simulink library "CryoDetLibCMB"  (R2016b)
settings: Solver=VariableStepAuto  StartTime=0.0  StopTime=10.0  RelTol=1e-3
undefined symbols (not defined in the file): Fclk, xlipgetpartsetting
libraries: xbsIndex_r4 x329, CryoDetLibCMB x20, CryoDetLib x2, simulink x1
(part 1 of 3)
settings Model: Creator=ssmith  LastModifiedBy=ssmith

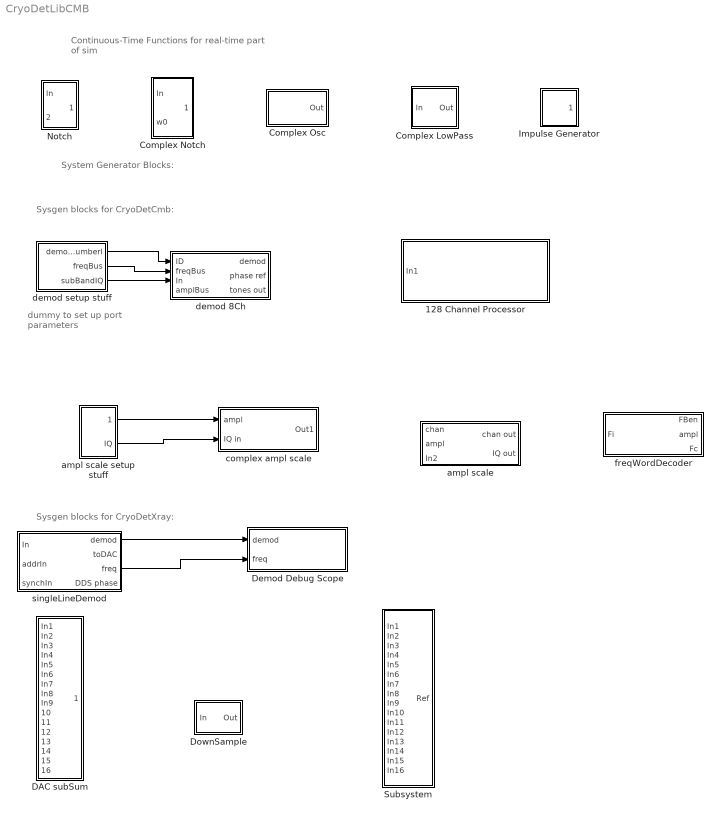
== system CryoDetLibCMB ==
  note: dummy to set up port parameters
  note: Sysgen blocks for CryoDetXray:
  note: Continuous-Time Functions
      | for real-time part of sim
  note: System Generator Blocks:
  note: Sysgen blocks for CryoDetCmb:
  128 Channel Processor : Subsystem
  Complex LowPass : Subsystem  mask{num=0, den=0}
  Complex Notch : Subsystem  mask(Complex Notch Filter){Q=10, depth=1, Q1=10, depth1=1, Q2=10, depth2=1}
      mask help: Specify w0, Q, and notch depth (1 is max depth, 0 is no notch)
      mask init:
      | Q1 = Q
      | depth1 = depth
      | Q2 = Q
      | depth2 = depth
      mask TypeOptions Q1: Notch1/Q
      mask TypeOptions depth1: Notch1/depth
      mask TypeOptions Q2: Notch2/Q
      mask TypeOptions depth2: Notch2/depth
  Complex Osc : Subsystem  mask{Freq=40e6, Ampl=0.2}
  DAC subSum : Subsystem
  Demod Debug Scope : Subsystem
  DownSample : Subsystem
  Impulse Generator : Subsystem  mask(Impulse Generator){Impulse=0, width=0, Period=0, delay=0}
      mask help:
      | Generate an psuedo-impulse via a rectangular pulse of amplitude given impulse/width so time intagral is impulse
      | repeating at period given by parameter Period starting at time "delay"
  Notch : Subsystem  mask(Notch filter){Q=10, depth=1}
      mask help:
      | Continuous-time notch filter acting in input with input parameters:
      | w0	center frequency
      | Q	center frequency/bandwidth
      | depth	depth of notch: 0==> no notch, 1 ==> deep notch
  Subsystem : Subsystem
  ampl scale : Subsystem
  ampl scale setup stuff : Subsystem
  complex ampl scale : Subsystem
  demod 8Ch : Subsystem
  demod setup stuff : Subsystem
  freqWordDecoder : Subsystem
  singleLineDemod : Subsystem
  wires:
  singleLineDemod/3(freq) -> Demod Debug Scope/2(freq)
  singleLineDemod/1(demod) -> Demod Debug Scope/1(demod)
  demod setup stuff/3(subBandIQ) -> demod 8Ch/3(In)
  demod setup stuff/1(demod numberl) -> demod 8Ch/1(ID)
  demod setup stuff/2(freqBus) -> demod 8Ch/2(freqBus)
  ampl scale setup stuff/1(ampl) -> complex ampl scale/1(ampl)
  ampl scale setup stuff/2(IQ) -> complex ampl scale/2(IQ in)

== system CryoDetLibCMB/128 Channel Processor ==
  note: dF using CORIDC rotation
      | added 11/14/17
  note: 128 Channel Processor
      | Contains baeband tone generator
      | demodulator
      | resonator frequency error estimator
      | loop filter
  In1 : Inport
  128 Channel Demodulator : Subsystem
  Loop Filter : Subsystem
  dF1 : Subsystem
  wires:
  In1/1 -> 128 Channel Demodulator/1(in)
  dF1/1(dF) -> Loop Filter/1(In2)
  128 Channel Demodulator/1(demod) -> dF1/1(demod)
  Loop Filter/1(Out2) -> 128 Channel Demodulator/2(freqBus)
  128 Channel Demodulator/2(phase ref out) -> dF1/2(ref phase)

== system CryoDetLibCMB/Complex LowPass ==
  note: Apply continuous-time transfer function given by num/den to complex continuous-time signal
  In : Inport
  Complex to Real-Imag : ComplexToRealImag
  Real-Imag to Complex : RealImagToComplex
  Transfer Fcn : TransferFcn  Numerator=num  Denominator=den
  Transfer Fcn1 : TransferFcn  Numerator=num  Denominator=den
  Out : Outport
  wires:
  Complex to Real-Imag/2 -> Transfer Fcn1/1
  Transfer Fcn1/1 -> Real-Imag to Complex/2
  In/1 -> Complex to Real-Imag/1
  Real-Imag to Complex/1 -> Out/1
  Transfer Fcn/1 -> Real-Imag to Complex/1
  Complex to Real-Imag/1 -> Transfer Fcn/1

== system CryoDetLibCMB/Complex Notch ==
  In : Inport
  w0 : Inport  Port=2
  Complex to Real-Imag : ComplexToRealImag
  Notch1 : CryoDetLib/Notch  Q=Q1  depth=depth1
  Notch2 : CryoDetLib/Notch  Q=Q2  depth=depth2
  Real-Imag to Complex : RealImagToComplex
  Out : Outport
  wires:
  Complex to Real-Imag/2 -> Notch2/1
  Notch2/1 -> Real-Imag to Complex/2
  In/1 -> Complex to Real-Imag/1
  Real-Imag to Complex/1 -> Out/1
  Notch1/1 -> Real-Imag to Complex/1
  w0/1 -> Notch2/2, Notch1/2
  Complex to Real-Imag/1 -> Notch1/1

== system CryoDetLibCMB/Complex Osc ==
  Cosine : Sin  Amplitude=Ampl  Frequency=2*pi*Freq  Phase=pi/2  SampleTime=0
  Real-Imag to Complex : RealImagToComplex
  Sine : Sin  Amplitude=Ampl  Frequency=2*pi*Freq  SampleTime=0
  Out : Outport
  wires:
  Real-Imag to Complex/1 -> Out/1
  Cosine/1 -> Real-Imag to Complex/1
  Sine/1 -> Real-Imag to Complex/2

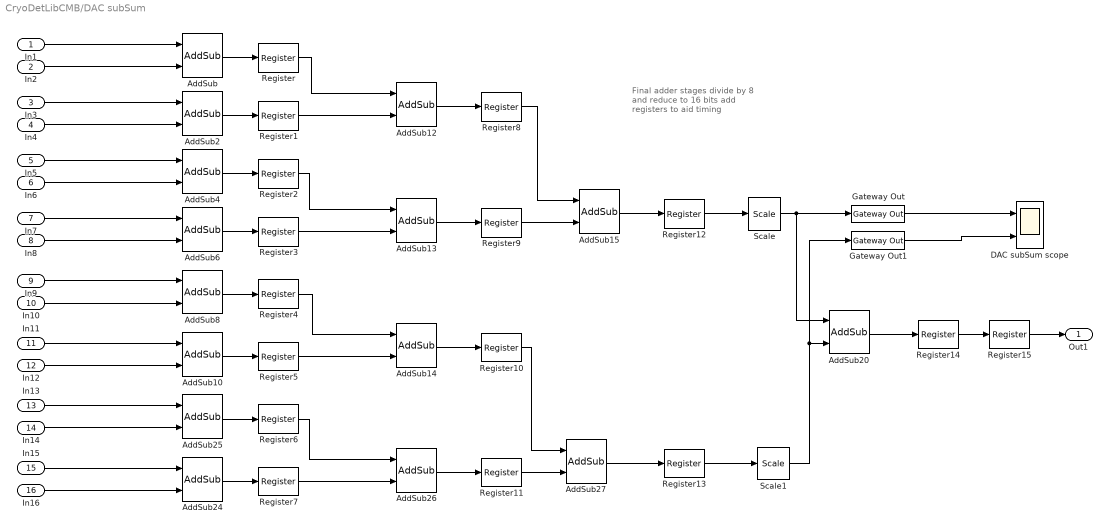
== system CryoDetLibCMB/DAC subSum ==
  note: Final adder stages
      | divide by 8
      | and reduce to 16 bits
      | add registers to aid timing
  In1 : Inport
  In2 : Inport  Port=2
  In3 : Inport  Port=3
  In4 : Inport  Port=4
  In5 : Inport  Port=5
  In6 : Inport  Port=6
  In7 : Inport  Port=7
  In8 : Inport  Port=8
  In9 : Inport  Port=9
  In10 : Inport  Port=10
  In11 : Inport  Port=11
  In12 : Inport  Port=12
  In13 : Inport  Port=13
  In14 : Inport  Port=14
  In15 : Inport  Port=15
  In16 : Inport  Port=16
  AddSub{,2,4,6,8,10,12..15,24..27} (14 alike) : xbsIndex_r4/AddSub  mode=Addition  use_carryin=off  use_carryout=off  en=off  latency=3  precision=User Defined  arith_type="Signed  (2's comp)"  n_bits=20  bin_pt=15  quantization=Truncate  overflow=Wrap  use_behavioral_HDL=off  hw_selection=Fabric  pipelined=off  dbl_ovrd=off  block_type=addsub
  AddSub20 : xbsIndex_r4/AddSub  mode=Addition  use_carryin=off  use_carryout=off  en=off  latency=3  precision=User Defined  arith_type="Signed  (2's comp)"  n_bits=16  bin_pt=15  quantization="Round  (unbiased: +/- Inf)"  overflow=Saturate  use_behavioral_HDL=off  hw_selection=Fabric  pipelined=off  dbl_ovrd=off  block_type=addsub
  DAC subSum scope : Scope  NumInputPorts=2
  Gateway Out : xbsIndex_r4/Gateway Out  inherit_from_input=off  hdl_port=off  rows=1  columns=1  UseAsDAC=off  DACChannel='1'  interface=None  automatic_assignment=on  address_offset=hex2dec('00')  intf_name=''  intf_description=''  timing_constraint=None  locs_specified=off  LOCs={}  io_standard={}  block_type=gatewayout
  Gateway Out1 : xbsIndex_r4/Gateway Out  inherit_from_input=off  hdl_port=off  rows=1  columns=1  UseAsDAC=off  DACChannel='1'  interface=None  automatic_assignment=on  address_offset=hex2dec('00')  intf_name=''  intf_description=''  timing_constraint=None  locs_specified=off  LOCs={}  io_standard={}  block_type=gatewayout
  Register{,1..15} (16 alike) : xbsIndex_r4/Register  init=0  rst=off  en=off  dbl_ovrd=off  block_type=register
  Scale : xbsIndex_r4/Scale  scale_factor=-3  dbl_ovrd=off  block_type=scale
  Scale1 : xbsIndex_r4/Scale  scale_factor=-3  dbl_ovrd=off  block_type=scale
  Out1 : Outport
  wires:
  AddSub20/1 -> Register14/1
  AddSub/1 -> Register/1
  AddSub2/1 -> Register1/1
  AddSub4/1 -> Register2/1
  AddSub6/1 -> Register3/1
  AddSub8/1 -> Register4/1
  AddSub10/1 -> Register5/1
  AddSub12/1 -> Register8/1
  AddSub13/1 -> Register9/1
  AddSub15/1 -> Register12/1
  In1/1 -> AddSub/1
  Scale/1 -> Gateway Out/1, AddSub20/1
  Scale1/1 -> Gateway Out1/1, AddSub20/2
  AddSub25/1 -> Register6/1
  AddSub24/1 -> Register7/1
  AddSub14/1 -> Register10/1
  AddSub27/1 -> Register13/1
  AddSub26/1 -> Register11/1
  In16/1 -> AddSub24/2
  In15/1 -> AddSub24/1
  In14/1 -> AddSub25/2
  In13/1 -> AddSub25/1
  In12/1 -> AddSub10/2
  In11/1 -> AddSub10/1
  In10/1 -> AddSub8/2
  In9/1 -> AddSub8/1
  In7/1 -> AddSub6/1
  In6/1 -> AddSub4/2
  In5/1 -> AddSub4/1
  In4/1 -> AddSub2/2
  In3/1 -> AddSub2/1
  In2/1 -> AddSub/2
  In8/1 -> AddSub6/2
  Gateway Out1/1 -> DAC subSum scope/2
  Gateway Out/1 -> DAC subSum scope/1
  Register/1 -> AddSub12/1
  Register1/1 -> AddSub12/2
  Register2/1 -> AddSub13/1
  Register3/1 -> AddSub13/2
  Register4/1 -> AddSub14/1
  Register5/1 -> AddSub14/2
  Register6/1 -> AddSub26/1
  Register7/1 -> AddSub26/2
  Register8/1 -> AddSub15/1
  Register9/1 -> AddSub15/2
  Register10/1 -> AddSub27/1
  Register11/1 -> AddSub27/2
  Register12/1 -> Scale/1
  Register13/1 -> Scale1/1
  Register14/1 -> Register15/1
  Register15/1 -> Out1/1

== system CryoDetLibCMB/Demod Debug Scope ==
  note: Debug Demodulation
  demod : Inport
  freq : Inport  Port=2
  Complex to Magnitude-Angle : ComplexToMagnitudeAngle  Output=Magnitude
  Demux1 : Demux
  Gain : Gain  Gain=Fclk
  Gateway Out{1,3..6} (5 alike) : xbsIndex_r4/Gateway Out  inherit_from_input=off  hdl_port=off  rows=1  columns=1  UseAsDAC=off  DACChannel='1'  interface=None  automatic_assignment=on  address_offset=hex2dec('00')  intf_name=''  intf_description=''  timing_constraint=None  locs_specified=off  LOCs={}  io_standard={}  block_type=gatewayout
  Mux4 : Mux  Inputs=3
  Mux5 : Mux  Inputs=2
  Real-Imag to Complex : RealImagToComplex
  block downconverter Scope : Scope  NumInputPorts=3
  wires:
  demod/1 -> Demux1/1
  Demux1/1 -> Gateway Out3/1
  Demux1/2 -> Gateway Out4/1
  Demux1/3 -> Gateway Out5/1
  Demux1/4 -> Gateway Out6/1
  Gateway Out6/1 -> Mux5/2
  Gateway Out5/1 -> Mux5/1
  Gateway Out4/1 -> Mux4/2, Real-Imag to Complex/1
  Gateway Out3/1 -> Mux4/1, Real-Imag to Complex/2
  Mux4/1 -> block downconverter Scope/1
  Mux5/1 -> block downconverter Scope/2
  Complex to Magnitude-Angle/1 -> Mux4/3
  Real-Imag to Complex/1 -> Complex to Magnitude-Angle/1
  freq/1 -> Gateway Out1/1
  Gateway Out1/1 -> Gain/1
  Gain/1 -> block downconverter Scope/3

== system CryoDetLibCMB/DownSample ==
  note: DownSample with rate change given by Naxi
  In : Inport
  Down Sample : xbsIndex_r4/Down Sample  sample_ratio=Naxi  sample_phase="Last Value of Frame  (most efficient)"  en=off  rst=off  latency=1  dbl_ovrd=off  block_type=dsamp
  Register : xbsIndex_r4/Register  init=0  rst=off  en=off  dbl_ovrd=off  block_type=register
  Register1 : xbsIndex_r4/Register  init=0  rst=off  en=off  dbl_ovrd=off  block_type=register
  Out : Outport
  wires:
  Register/1 -> Register1/1
  In/1 -> Down Sample/1
  Down Sample/1 -> Register/1
  Register1/1 -> Out/1

== system CryoDetLibCMB/Impulse Generator ==
  note: Parameters are:
      | width:	 pulse width (seconds)
      | Impulse:	Area of pulse = Amplitude*width
      | Period:	Pulse repetition time (seconds)
      | delay:	start time of pulse (seconds)
  Pulse Generator1 : DiscretePulseGenerator  PulseType=Time based  Amplitude=Impulse/width  Period=Period  PulseWidth=100 * width/Period  PhaseDelay=delay
  Out1 : Outport
  wires:
  Pulse Generator1/1 -> Out1/1

== system CryoDetLibCMB/Notch ==
  note: Notch Filter with center angular frequency w0, finite Q, and notch depth
  In : Inport
  w0 : Inport  Port=2
  Gain : Gain  Gain=depth
  Gain1 : Gain  Gain=1/Q
  Integrator1 : Integrator
  Integrator4 : Integrator
  Product : Product
  Product1 : Product
  Sum1 : Sum  Inputs=++|
  Sum2 : Sum  Inputs=|+-
  Sum3 : Sum  Inputs=-+|
  out : Outport
  wires:
  Gain1/1 -> Gain/1, Sum1/1
  Sum2/1 -> Integrator1/1
  In/1 -> Sum2/1, Sum3/2
  w0/1 -> Product/1, Product1/1
  Integrator1/1 -> Product/2
  Product/1 -> Integrator4/1, Gain1/1
  Gain/1 -> Sum3/1
  Sum1/1 -> Sum2/2
  Sum3/1 -> out/1
  Product1/1 -> Sum1/2
  Integrator4/1 -> Product1/2

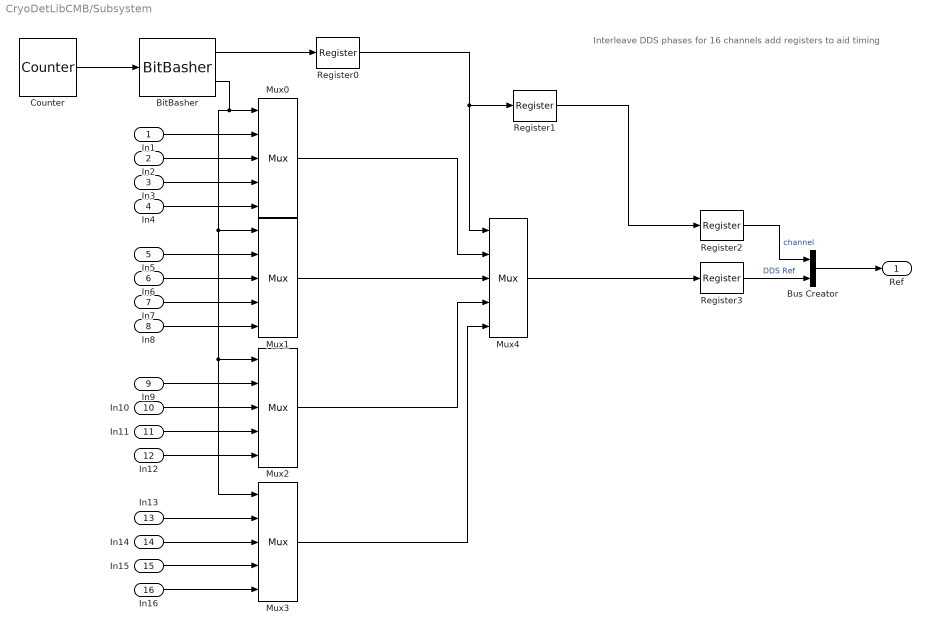
== system CryoDetLibCMB/Subsystem ==
  note: Interleave DDS phases for 16 channels
      | add registers to aid timing
  In1 : Inport
  In2 : Inport  Port=2
  In3 : Inport  Port=3
  In4 : Inport  Port=4
  In5 : Inport  Port=5
  In6 : Inport  Port=6
  In7 : Inport  Port=7
  In8 : Inport  Port=8
  In9 : Inport  Port=9
  In10 : Inport  Port=10
  In11 : Inport  Port=11
  In12 : Inport  Port=12
  In13 : Inport  Port=13
  In14 : Inport  Port=14
  In15 : Inport  Port=15
  In16 : Inport  Port=16
  BitBasher : xbsIndex_r4/BitBasher  bitexpr=|  display_expr=on  sr_1=hi  arith_type1=Unsigned  bin_pt1=0  sr_2=lo  arith_type2=Unsigned  bin_pt2=0  sr_3=3  arith_type3=Unsigned  bin_pt3=0  sr_4=4  arith_type4=Unsigned  bin_pt4=0  dbl_ovrd=off  block_type=bitbasher
      | hi = {in[3:2]}
      | lo = {in[1:0]}
  Bus Creator : BusCreator  Inputs=2
  Counter : xbsIndex_r4/Counter  cnt_type=Free Running  cnt_to=Inf  operation=Up  start_count=0  cnt_by_val=1  arith_type=Unsigned  n_bits=4  bin_pt=0  load_pin=off  rst=off  en=off  explicit_period=on  period=Tclk  use_behavioral_HDL=off  implementation=Fabric  dbl_ovrd=off  block_type=counter
  Mux{0..4} (5 alike) : xbsIndex_r4/Mux  inputs=4  en=off  latency=1  precision=Full  arith_type=Unsigned  n_bits=16  bin_pt=14  quantization=Truncate  overflow=Wrap  dbl_ovrd=off  block_type=mux
  Register{0..3} (4 alike) : xbsIndex_r4/Register  init=0  rst=off  en=off  dbl_ovrd=off  block_type=register
  Ref : Outport
  wires:
  In13/1 -> Mux3/2
  In6/1 -> Mux1/3
  Mux0/1 -> Mux4/2
  BitBasher/2 -> Mux1/1, Mux2/1, Mux3/1, Mux0/1
  In8/1 -> Mux1/5
  In10/1 -> Mux2/3
  In3/1 -> Mux0/4
  In14/1 -> Mux3/3
  BitBasher/1 -> Register0/1
  In9/1 -> Mux2/2
  In11/1 -> Mux2/4
  Mux1/1 -> Mux4/3
  In2/1 -> Mux0/3
  In15/1 -> Mux3/4
  In4/1 -> Mux0/5
  Mux3/1 -> Mux4/5
  In1/1 -> Mux0/2
  In5/1 -> Mux1/2
  In12/1 -> Mux2/5
  Register0/1 -> Register1/1, Mux4/1
  In7/1 -> Mux1/4
  Counter/1 -> BitBasher/1
  Mux2/1 -> Mux4/4
  Mux4/1 -> Register3/1
  In16/1 -> Mux3/5
  Register3/1 -> Bus Creator/2  "DDS Ref"
  Bus Creator/1 -> Ref/1
  Register2/1 -> Bus Creator/1  "channel"
  Register1/1 -> Register2/1

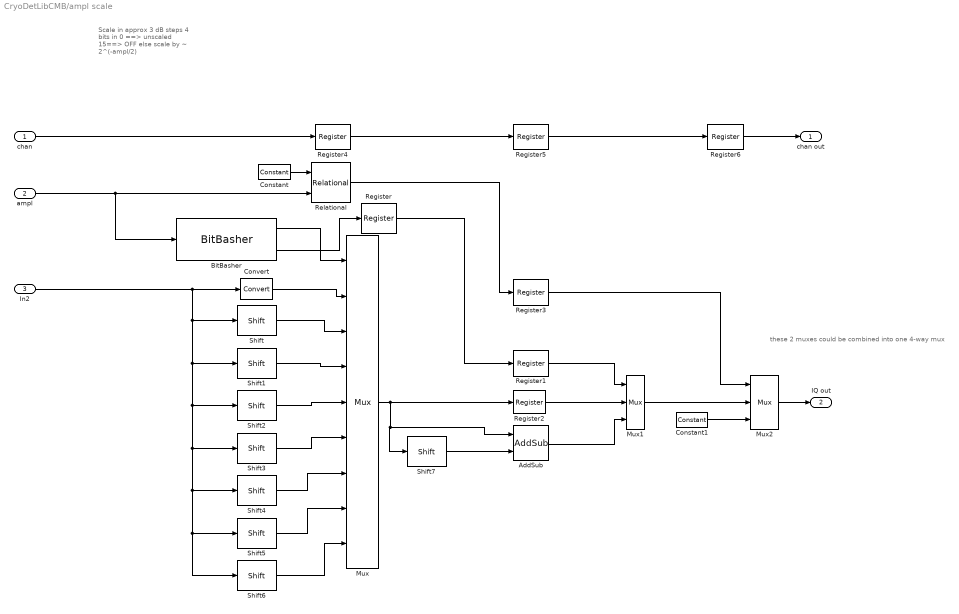
== system CryoDetLibCMB/ampl scale ==
  note: these 2 muxes could be combined into one 4-way mux
  note: Scale in approx 3 dB steps
      | 4 bits in
      | 0 ==> unscaled
      | 15==> OFF
      | else scale by ~ 2^(-ampl/2)
  chan : Inport
  ampl : Inport  Port=2
  In2 : Inport  Port=3
  AddSub : xbsIndex_r4/AddSub  mode=Subtraction  use_carryin=off  use_carryout=off  en=off  latency=1  precision=User Defined  arith_type=Unsigned  n_bits=18  bin_pt=16  quantization=Truncate  overflow=Wrap  use_behavioral_HDL=off  hw_selection=Fabric  pipelined=off  dbl_ovrd=off  block_type=addsub
  BitBasher : xbsIndex_r4/BitBasher  bitexpr=|  display_expr=on  sr_1=int  arith_type1=Unsigned  bin_pt1=0  sr_2=frac  arith_type2=Unsigned  bin_pt2=0  sr_3=3  arith_type3=Unsigned  bin_pt3=0  sr_4=4  arith_type4=Unsigned  bin_pt4=0  dbl_ovrd=off  block_type=bitbasher
      | int = {ampl[3:1]}
      | frac = {ampl[0:0]}
  Constant : xbsIndex_r4/Constant  const=15  gui_display_data_type=Fixed-point  arith_type=Unsigned  n_bits=4  bin_pt=0  preci_type=Single  exp_width=8  frac_width=24  explicit_period=off  period=1  equ=P=C  opselect=C  inp2=PCIN>>17  opr=+  inp1=P  carry=CIN  dbl_ovrd=off  block_type=constant
  Constant1 : xbsIndex_r4/Constant  const=0  gui_display_data_type=Fixed-point  arith_type=Signed (2's comp)  n_bits=18  bin_pt=16  preci_type=Single  exp_width=8  frac_width=24  explicit_period=off  period=1  equ=P=C  opselect=C  inp2=PCIN>>17  opr=+  inp1=P  carry=CIN  dbl_ovrd=off  block_type=constant
  Convert : xbsIndex_r4/Convert  gui_display_data_type=Fixed-point  arith_type="Signed  (2's comp)"  n_bits=18  bin_pt=16  float_type=Single  exp_bits=8  fraction_bits=24  quantization=Truncate  overflow=Wrap  en=off  latency=0  pipeline=off  dbl_ovrd=off  block_type=convert
  Mux : xbsIndex_r4/Mux  inputs=8  en=off  latency=1  precision=Full  arith_type=Unsigned  n_bits=16  bin_pt=14  quantization=Truncate  overflow=Wrap  dbl_ovrd=off  block_type=mux
  Mux1 : xbsIndex_r4/Mux  inputs=2  en=off  latency=0  precision=Full  arith_type=Unsigned  n_bits=16  bin_pt=14  quantization=Truncate  overflow=Wrap  dbl_ovrd=off  block_type=mux
  Mux2 : xbsIndex_r4/Mux  inputs=2  en=off  latency=1  precision=Full  arith_type=Unsigned  n_bits=16  bin_pt=14  quantization=Truncate  overflow=Wrap  dbl_ovrd=off  block_type=mux
  Register{,1..6} (7 alike) : xbsIndex_r4/Register  init=0  rst=off  en=off  dbl_ovrd=off  block_type=register
  Relational : xbsIndex_r4/Relational  mode=a=b  op_type=Bool  en=off  latency=1  dbl_ovrd=off  block_type=relational
  Shift : xbsIndex_r4/Shift  shift_dir=Right  shift_bits=1  en=off  latency=0  precision=User Defined  arith_type="Signed  (2's comp)"  n_bits=18  bin_pt=16  quantization=Truncate  overflow=Wrap  dbl_ovrd=off  block_type=shift
  Shift1 : xbsIndex_r4/Shift  shift_dir=Right  shift_bits=2  en=off  latency=0  precision=User Defined  arith_type="Signed  (2's comp)"  n_bits=18  bin_pt=16  quantization=Truncate  overflow=Wrap  dbl_ovrd=off  block_type=shift
  Shift2 : xbsIndex_r4/Shift  shift_dir=Right  shift_bits=3  en=off  latency=0  precision=User Defined  arith_type="Signed  (2's comp)"  n_bits=18  bin_pt=16  quantization=Truncate  overflow=Wrap  dbl_ovrd=off  block_type=shift
  Shift3 : xbsIndex_r4/Shift  shift_dir=Right  shift_bits=4  en=off  latency=0  precision=User Defined  arith_type="Signed  (2's comp)"  n_bits=18  bin_pt=16  quantization=Truncate  overflow=Wrap  dbl_ovrd=off  block_type=shift
  Shift4 : xbsIndex_r4/Shift  shift_dir=Right  shift_bits=5  en=off  latency=0  precision=User Defined  arith_type="Signed  (2's comp)"  n_bits=18  bin_pt=16  quantization=Truncate  overflow=Wrap  dbl_ovrd=off  block_type=shift
  Shift5 : xbsIndex_r4/Shift  shift_dir=Right  shift_bits=6  en=off  latency=0  precision=User Defined  arith_type="Signed  (2's comp)"  n_bits=18  bin_pt=16  quantization=Truncate  overflow=Wrap  dbl_ovrd=off  block_type=shift
  Shift6 : xbsIndex_r4/Shift  shift_dir=Right  shift_bits=7  en=off  latency=0  precision=User Defined  arith_type="Signed  (2's comp)"  n_bits=18  bin_pt=16  quantization=Truncate  overflow=Wrap  dbl_ovrd=off  block_type=shift
  Shift7 : xbsIndex_r4/Shift  shift_dir=Right  shift_bits=2  en=off  latency=0  precision=User Defined  arith_type="Signed  (2's comp)"  n_bits=18  bin_pt=16  quantization=Truncate  overflow=Wrap  dbl_ovrd=off  block_type=shift
  chan out : Outport
  IQ out : Outport  Port=2
  wires:
  Shift1/1 -> Mux/4
  Shift/1 -> Mux/3
  Shift2/1 -> Mux/5
  Shift3/1 -> Mux/6
  Shift4/1 -> Mux/7
  Shift5/1 -> Mux/8
  Shift6/1 -> Mux/9
  Mux/1 -> AddSub/1, Shift7/1, Register2/1
  Shift7/1 -> AddSub/2
  AddSub/1 -> Mux1/3
  ampl/1 -> BitBasher/1, Relational/2
  BitBasher/1 -> Mux/1
  BitBasher/2 -> Register/1
  Constant/1 -> Relational/1
  In2/1 -> Shift/1, Shift3/1, Shift4/1, Shift5/1, Shift6/1, Shift2/1, Shift1/1, Convert/1
  Register/1 -> Register1/1
  Register1/1 -> Mux1/1
  Register2/1 -> Mux1/2
  Relational/1 -> Register3/1
  Mux1/1 -> Mux2/2
  Mux2/1 -> IQ out/1
  Constant1/1 -> Mux2/3
  Register3/1 -> Mux2/1
  Convert/1 -> Mux/2
  chan/1 -> Register4/1
  Register4/1 -> Register5/1
  Register5/1 -> Register6/1
  Register6/1 -> chan out/1

== system CryoDetLibCMB/ampl scale setup stuff ==
  Bus Creator : BusCreator  Inputs=3
  Constant : xbsIndex_r4/Constant  const=7  gui_display_data_type=Fixed-point  arith_type=Unsigned  n_bits=3  bin_pt=0  preci_type=Single  exp_width=8  frac_width=24  explicit_period=off  period=1  equ=P=C  opselect=C  inp2=PCIN>>17  opr=+  inp1=P  carry=CIN  dbl_ovrd=off  block_type=constant
  Constant1 : xbsIndex_r4/Constant  const=3  gui_display_data_type=Fixed-point  arith_type=Unsigned  n_bits=3  bin_pt=0  preci_type=Single  exp_width=8  frac_width=24  explicit_period=off  period=1  equ=P=C  opselect=C  inp2=PCIN>>17  opr=+  inp1=P  carry=CIN  dbl_ovrd=off  block_type=constant
  Constant2 : xbsIndex_r4/Constant  const=0.1234  gui_display_data_type=Fixed-point  arith_type=Signed (2's comp)  n_bits=16  bin_pt=14  preci_type=Single  exp_width=8  frac_width=24  explicit_period=off  period=1  equ=P=C  opselect=C  inp2=PCIN>>17  opr=+  inp1=P  carry=CIN  dbl_ovrd=off  block_type=constant
  Constant3 : xbsIndex_r4/Constant  const=05678  gui_display_data_type=Fixed-point  arith_type=Signed (2's comp)  n_bits=16  bin_pt=14  preci_type=Single  exp_width=8  frac_width=24  explicit_period=off  period=1  equ=P=C  opselect=C  inp2=PCIN>>17  opr=+  inp1=P  carry=CIN  dbl_ovrd=off  block_type=constant
  ampl : Outport
  IQ : Outport  Port=2
  wires:
  Bus Creator/1 -> IQ/1
  Constant/1 -> Bus Creator/1  "band"
  Constant3/1 -> Bus Creator/3  "I"
  Constant2/1 -> Bus Creator/2  "Q"
  Constant1/1 -> ampl/1

== system CryoDetLibCMB/complex ampl scale ==
  ampl : Inport
  IQ in : Inport  Port=2
  Bus Creator : BusCreator  Inputs=3
  Bus Selector : BusSelector  OutputSignals=band,Q,I
  Terminator : Terminator
  ampl scale : CryoDetLibCMB/ampl scale
  ampl scale1 : CryoDetLibCMB/ampl scale
  Out1 : Outport
  wires:
  IQ in/1 -> Bus Selector/1
  Bus Creator/1 -> Out1/1
  ampl/1 -> ampl scale/2, ampl scale1/2
  ampl scale/1 -> Bus Creator/1  "band"
  ampl scale/2 -> Bus Creator/2  "Q"
  ampl scale1/2 -> Bus Creator/3  "I"
  Bus Selector/1 -> ampl scale1/1, ampl scale/1  "<band>"
  Bus Selector/3 -> ampl scale1/3  "<I>"
  Bus Selector/2 -> ampl scale/3  "<Q>"
  ampl scale1/1 -> Terminator/1

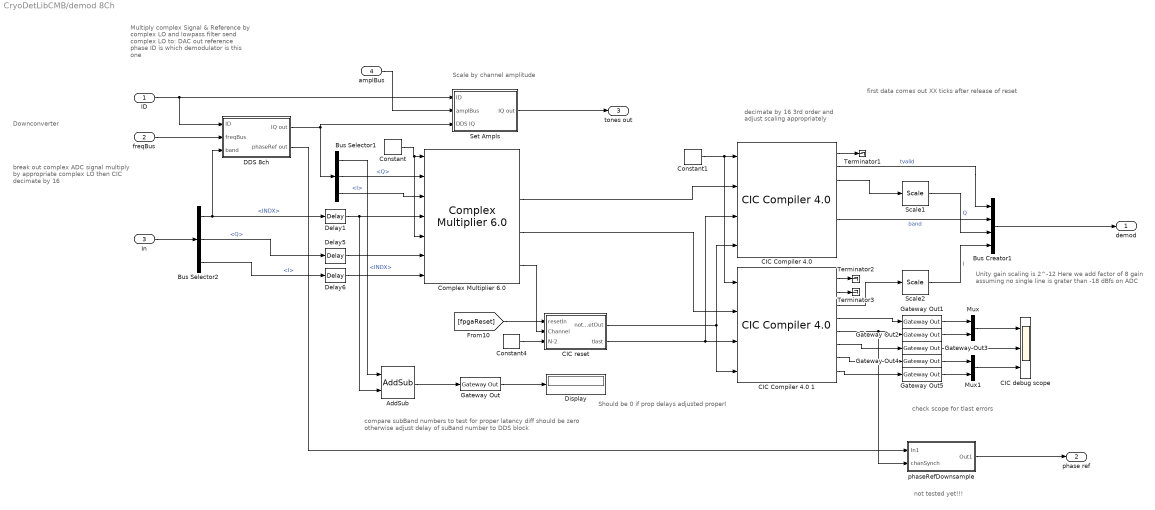
== system CryoDetLibCMB/demod 8Ch ==
  note: Scale by channel amplitude
  note: not tested yet!!!
  note: check scope for tlast errors
  note: Unity gain scaling is 2^-12
      | Here we add factor of 8 gain
      | assuming no single line is grater than -18 dBfs on ADC
  note: Should be 0 if prop delays adjusted properl
  note: compare subBand numbers to test for proper latency
      | diff should be zero otherwise adjust delay of suBand number to DDS block
  note: decimate by 16 3rd order
      | and adjust scaling appropriately
  note: Downconverter
  note: Multiply complex Signal & Reference
      | by complex LO and lowpass filter
      | send complex LO to:
      | 	DAC out
      | 	reference phase
      | ID is which demodulator is this one
  note: break out complex ADC signal
      | multiply by appropriate complex LO
      | then CIC decimate by 16
  note: first data comes out XX ticks after release of reset
  ID : Inport
  freqBus : Inport  Port=2
  In : Inport  Port=3
  amplBus : Inport  Port=4
  AddSub : xbsIndex_r4/AddSub  mode=Subtraction  use_carryin=off  use_carryout=off  en=off  latency=1  precision=User Defined  arith_type="Signed  (2's comp)"  n_bits=3  bin_pt=0  quantization=Truncate  overflow=Wrap  use_behavioral_HDL=off  hw_selection=Fabric  pipelined=off  dbl_ovrd=off  block_type=addsub
  Bus Creator1 : BusCreator  Inputs=4
  Bus Selector1 : BusSelector  OutputSignals=INDX,Q,I
  Bus Selector2 : BusSelector  OutputSignals=INDX,Q,I
  "CIC Compiler 4.0 " : xbsIndex_r4/CIC Compiler 4.0   filter_type=Decimation  number_of_stages=3  differential_delay=1  number_of_channels=8  sample_rate_changes=Fixed  fixed_or_initial_rate=16  minimum_rate=16  maximum_rate=16  ratespecification=Sample_Period  sampleperiod=1  hardwareoversamplingrate=1  quantization=Truncation  output_data_width=20  use_xtreme_dsp_slice=off  use_streaming_interface=on  has_aclken=off  has_aresetn=on  has_dout_tready=off  trim_axipin_name=on  gui_behaviour=Sysgen_GUI  input_data_width=18  ip_name=CIC Compiler  ip_version=4.0  dsptool_ready=true  wrapper_available=true  port_translation_map={ 'aclken' => 'en', 'aresetn' => 'rst' }  ipcore_xco_need_fpga_part=true  ipcore_verbose=false  block_type=cic_compiler_v4_0
  CIC Compiler 4.0 1 : xbsIndex_r4/CIC Compiler 4.0   filter_type=Decimation  number_of_stages=3  differential_delay=1  number_of_channels=8  sample_rate_changes=Fixed  fixed_or_initial_rate=16  minimum_rate=16  maximum_rate=16  ratespecification=Sample_Period  sampleperiod=1  hardwareoversamplingrate=1  quantization=Truncation  output_data_width=20  use_xtreme_dsp_slice=off  use_streaming_interface=on  has_aclken=off  has_aresetn=on  has_dout_tready=off  trim_axipin_name=on  gui_behaviour=Sysgen_GUI  input_data_width=18  ip_name=CIC Compiler  ip_version=4.0  dsptool_ready=true  wrapper_available=true  port_translation_map={ 'aclken' => 'en', 'aresetn' => 'rst' }  ipcore_xco_need_fpga_part=true  ipcore_verbose=false  block_type=cic_compiler_v4_0
  CIC debug scope : Scope  NumInputPorts=3
  CIC reset : Subsystem
  "Complex Multiplier 6.0 " : xbsIndex_r4/Complex Multiplier 6.0   hasatlast=off  hasatuser=on  atuserwidth=3  hasbtlast=off  hasbtuser=off  btuserwidth=1  multtype=Use_Mults  optimizegoal=Resources  flowcontrol=NonBlocking  outputwidth=18  roundmode=Truncate  hasctrltlast=off  hasctrltuser=off  ctrltuserwidth=1  outtlastbehv=Null  latencyconfig=Manual  minimumlatency=6  aclken=off  aresetn=off  trim_axipin_name=on  simulation_type=hybrid_sim  simulation_model=sysgen:cmpy_v6_0  data_path_portlist={ 's_axis_a_tdata_real', 's_axis_a_tdata_imag', 's_axis_b_tdata_real', 's_axis_b_tdata_imag', 's_axis_ctrl_tdata_rounding_bit', 'm_axis_dout_tdata_real', 'm_axis_dout_tdata_imag' }  aportwidth=63  bportwidth=63  ip_name=Complex Multiplier  ip_version=6.0  dsptool_ready=true  ipcore_usecache=true  ipcore_useipmodelcache=true  ipcore_verbose=false  ipcore_latency_parameter='minimumlatency'  wrapper_available=true  port_translation_map={ 'aclken' => 'en', 'aresetn' => 'rst'}  block_type=cmpy_v6_0
  Constant : xbsIndex_r4/Constant  const=1  gui_display_data_type=Boolean  arith_type=Boolean  n_bits=16  bin_pt=14  preci_type=Single  exp_width=8  frac_width=24  explicit_period=off  period=1  equ=P=C  opselect=C  inp2=PCIN>>17  opr=+  inp1=P  carry=CIN  dbl_ovrd=off  block_type=constant
  Constant1 : xbsIndex_r4/Constant  const=1  gui_display_data_type=Boolean  arith_type=Boolean  n_bits=16  bin_pt=14  preci_type=Single  exp_width=8  frac_width=24  explicit_period=off  period=1  equ=P=C  opselect=C  inp2=PCIN>>17  opr=+  inp1=P  carry=CIN  dbl_ovrd=off  block_type=constant
  Constant4 : xbsIndex_r4/Constant  const=14  gui_display_data_type=Fixed-point  arith_type=Unsigned  n_bits=4  bin_pt=0  preci_type=Single  exp_width=8  frac_width=24  explicit_period=off  period=1  equ=P=C  opselect=C  inp2=PCIN>>17  opr=+  inp1=P  carry=CIN  dbl_ovrd=off  block_type=constant
  DDS 8ch : Subsystem
  Delay1 : xbsIndex_r4/Delay  rst=off  infoeditControl=Selection of Reset will increase slice count due to use of real FFs and instead of SRLs  en=off  latency=1  reg_retiming=on  dbl_ovrd=off  block_type=delay
  Delay5 : xbsIndex_r4/Delay  rst=off  infoeditControl=Selection of Reset will increase slice count due to use of real FFs and instead of SRLs  en=off  latency=1  reg_retiming=on  dbl_ovrd=off  block_type=delay
  Delay6 : xbsIndex_r4/Delay  rst=off  infoeditControl=Selection of Reset will increase slice count due to use of real FFs and instead of SRLs  en=off  latency=1  reg_retiming=on  dbl_ovrd=off  block_type=delay
  Display : Display
  Gateway Out{,1..5} (6 alike) : xbsIndex_r4/Gateway Out  inherit_from_input=off  hdl_port=off  rows=1  columns=1  UseAsDAC=off  DACChannel='1'  interface=None  automatic_assignment=on  address_offset=hex2dec('00')  intf_name=''  intf_description=''  timing_constraint=None  locs_specified=off  LOCs={}  io_standard={}  block_type=gatewayout
  Mux : Mux  Inputs=2
  Mux1 : Mux  Inputs=2
  Scale1 : xbsIndex_r4/Scale  scale_factor=-9  dbl_ovrd=off  block_type=scale
  Scale2 : xbsIndex_r4/Scale  scale_factor=-9  dbl_ovrd=off  block_type=scale
  Set Ampls : Subsystem
  Terminator1 : Terminator
  Terminator2 : Terminator
  Terminator3 : Terminator
  phaseRefDownsample : Subsystem
  demod : Outport
  phase ref : Outport  Port=2
  tones out : Outport  Port=3
  wires:
  In/1 -> Bus Selector2/1
  Bus Selector1/2 -> "Complex Multiplier 6.0 "/2  "<Q>"
  Bus Selector1/3 -> "Complex Multiplier 6.0 "/3  "<I>"
  "Complex Multiplier 6.0 "/2 -> "CIC Compiler 4.0 "/2
  "CIC Compiler 4.0 "/3 -> Scale1/1
  CIC Compiler 4.0 1/3 -> Scale2/1
  "CIC Compiler 4.0 "/1 -> Terminator1/1
  CIC Compiler 4.0 1/1 -> Terminator2/1
  CIC Compiler 4.0 1/2 -> Terminator3/1
  "Complex Multiplier 6.0 "/3 -> CIC Compiler 4.0 1/2
  Constant/1 -> "Complex Multiplier 6.0 "/5, "Complex Multiplier 6.0 "/1
  freqBus/1 -> DDS 8ch/2(freqBus)
  Bus Selector2/1 -> Delay1/1, DDS 8ch/3(band)  "<INDX>"
  Bus Selector2/2 -> Delay5/1  "<Q>"
  Bus Selector2/3 -> Delay6/1  "<I>"
  DDS 8ch/1(IQ out) -> Set Ampls/3(DDS IQ), Bus Selector1/1
  Delay1/1 -> AddSub/2, "Complex Multiplier 6.0 "/4
  Delay5/1 -> "Complex Multiplier 6.0 "/6
  Delay6/1 -> "Complex Multiplier 6.0 "/7
  Bus Selector1/1 -> AddSub/1  "<INDX>"
  AddSub/1 -> Gateway Out/1
  Gateway Out/1 -> Display/1
  Constant1/1 -> CIC Compiler 4.0 1/1, "CIC Compiler 4.0 "/1
  Constant4/1 -> CIC reset/3(N-2)
  [fpgaReset] -> CIC reset/1(resetIn)
  CIC reset/1(notResetOut) -> "CIC Compiler 4.0 "/4, CIC Compiler 4.0 1/4
  "Complex Multiplier 6.0 "/4 -> CIC reset/2(Channel)
  CIC reset/2(tlast) -> CIC Compiler 4.0 1/3, "CIC Compiler 4.0 "/3
  "CIC Compiler 4.0 "/6 -> Bus Creator1/2  "band"
  Scale1/1 -> Bus Creator1/3  "Q"
  Scale2/1 -> Bus Creator1/4  "I"
  CIC Compiler 4.0 1/4 -> Gateway Out1/1
  CIC Compiler 4.0 1/5 -> phaseRefDownsample/2(chanSynch), Gateway Out2/1
  CIC Compiler 4.0 1/6 -> Gateway Out3/1
  CIC Compiler 4.0 1/7 -> Gateway Out4/1
  CIC Compiler 4.0 1/8 -> Gateway Out5/1
  Gateway Out2/1 -> Mux/2
  Gateway Out1/1 -> Mux/1
  Gateway Out5/1 -> Mux1/2
  Gateway Out4/1 -> Mux1/1
  Mux/1 -> CIC debug scope/1
  Gateway Out3/1 -> CIC debug scope/2
  Mux1/1 -> CIC debug scope/3
  "CIC Compiler 4.0 "/2 -> Bus Creator1/1  "tvalid"
  DDS 8ch/2(phaseRef out) -> phaseRefDownsample/1(In1)
  phaseRefDownsample/1(Out1) -> phase ref/1
  ID/1 -> Set Ampls/1(ID), DDS 8ch/1(ID)
  amplBus/1 -> Set Ampls/2(amplBus)
  Bus Creator1/1 -> demod/1
  Set Ampls/1(IQ out) -> tones out/1

== system CryoDetLibCMB/demod setup stuff ==
  Bus Creator : BusCreator  Inputs=3
  Bus Creator1 : BusCreator  Inputs=3
  Counter Free-Running1 : simulink/Sources/Counter Free-Running  NumBits=3  tsamp=Tclk
  I : xbsIndex_r4/Constant  const=1  gui_display_data_type=Fixed-point  arith_type=Signed (2's comp)  n_bits=25  bin_pt=24  preci_type=Single  exp_width=8  frac_width=24  explicit_period=on  period=Tclk  equ=P=C  opselect=C  inp2=PCIN>>17  opr=+  inp1=P  carry=CIN  dbl_ovrd=off  block_type=constant
  Ndemod : xbsIndex_r4/Constant  const=15  gui_display_data_type=Fixed-point  arith_type=Unsigned  n_bits=4  bin_pt=0  preci_type=Single  exp_width=8  frac_width=24  explicit_period=off  period=1  equ=P=C  opselect=C  inp2=PCIN>>17  opr=+  inp1=P  carry=CIN  dbl_ovrd=off  block_type=constant
  Q : xbsIndex_r4/Constant  const=0  gui_display_data_type=Fixed-point  arith_type=Signed (2's comp)  n_bits=25  bin_pt=24  preci_type=Single  exp_width=8  frac_width=24  explicit_period=on  period=Tclk  equ=P=C  opselect=C  inp2=PCIN>>17  opr=+  inp1=P  carry=CIN  dbl_ovrd=off  block_type=constant
  demod # : xbsIndex_r4/Constant  const=15  gui_display_data_type=Fixed-point  arith_type=Unsigned  n_bits=4  bin_pt=0  preci_type=Single  exp_width=8  frac_width=24  explicit_period=off  period=1  equ=P=C  opselect=C  inp2=PCIN>>17  opr=+  inp1=P  carry=CIN  dbl_ovrd=off  block_type=constant
  freq2 : xbsIndex_r4/Constant  const=0.12345 * 2^24  gui_display_data_type=Fixed-point  arith_type=Unsigned  n_bits=24  bin_pt=0  preci_type=Single  exp_width=8  frac_width=24  explicit_period=on  period=Tclk  equ=P=C  opselect=C  inp2=PCIN>>17  opr=+  inp1=P  carry=CIN  dbl_ovrd=off  block_type=constant
  subCh : xbsIndex_r4/Constant  const=7  gui_display_data_type=Fixed-point  arith_type=Unsigned  n_bits=3  bin_pt=0  preci_type=Single  exp_width=8  frac_width=24  explicit_period=off  period=1  equ=P=C  opselect=C  inp2=PCIN>>17  opr=+  inp1=P  carry=CIN  dbl_ovrd=off  block_type=constant
  demod numberl : Outport
  freqBus : Outport  Port=2
  subBandIQ : Outport  Port=3
  wires:
  Bus Creator/1 -> freqBus/1
  demod #/1 -> demod numberl/1
  freq2/1 -> Bus Creator/3  "freq"
  subCh/1 -> Bus Creator/1  "band"
  Ndemod/1 -> Bus Creator/2  "chan"
  Bus Creator1/1 -> subBandIQ/1
  Counter Free-Running1/1 -> Bus Creator1/1  "INDX"
  Q/1 -> Bus Creator1/2  "Q"
  I/1 -> Bus Creator1/3  "I"

== system CryoDetLibCMB/freqWordDecoder ==
  Fi : Inport
  BitBasher : xbsIndex_r4/BitBasher  bitexpr=|  display_expr=on  sr_1=FBen  arith_type1=Unsigned  bin_pt1=0  sr_2=ampl  arith_type2=Unsigned  bin_pt2=0  sr_3=Finit  arith_type3=Unsigned  bin_pt3=23  sr_4=4  arith_type4=Unsigned  bin_pt4=0  dbl_ovrd=off  block_type=bitbasher
      | FBen = {freqWord[31:31]}
      | ampl = {freqWord[27:24]}
      | Finit = {freqWord[23:0]}
  FBen : Outport
  ampl : Outport  Port=2
  Fc : Outport  Port=3
  wires:
  BitBasher/2 -> ampl/1
  BitBasher/3 -> Fc/1
  BitBasher/1 -> FBen/1
  Fi/1 -> BitBasher/1

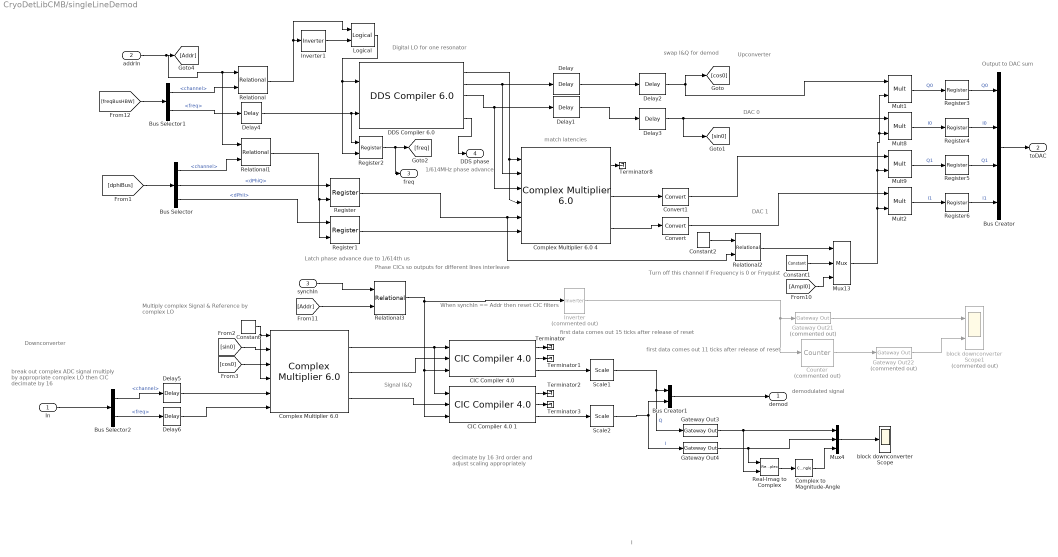
== system CryoDetLibCMB/singleLineDemod ==
  note: swap I&Q for demod
  note: Output to DAC sum
  note: decimate by 16 3rd order
      | and adjust scaling appropriately
  note: When synchIn == Addr then reset CIC filters
  note: Turn off this channel if Frequency is 0 or Fnyquist
  note: first data comes out 15 ticks after release of reset
  note: Latch phase advance due to 1/614th us
  note: I
  note: DAC 1
  note: DAC 0
  note: Downconverter
  note: demodulated signal
  note: Phase CICs so outputs for different lines interleave
  note: Signal I&Q
  note: Multiply complex Signal & Reference
      | by complex LO
  note: match latencies
  note: 1/614MHz
      | phase advance
  note: break out complex ADC signal
      | multiply by appropriate complex LO
      | then CIC decimate by 16
  note: Digital LO for one resonator
  note: Upconverter
  note: first data comes out 11 ticks after release of reset
  In : Inport
  addrIn : Inport  Port=2
  synchIn : Inport  Port=3
  Bus Creator : BusCreator  Inputs=4
  Bus Creator1 : BusCreator  Inputs=2
  Bus Selector : BusSelector  OutputSignals=channel,dPhiQ,dPhiI
  Bus Selector1 : BusSelector  OutputSignals=channel,freq
  Bus Selector2 : BusSelector  OutputSignals=channel,freq
  "CIC Compiler 4.0 " : xbsIndex_r4/CIC Compiler 4.0   filter_type=Decimation  number_of_stages=3  differential_delay=1  number_of_channels=1  sample_rate_changes=Fixed  fixed_or_initial_rate=16  minimum_rate=16  maximum_rate=16  ratespecification=Sample_Period  sampleperiod=1  hardwareoversamplingrate=1  quantization=Truncation  output_data_width=20  use_xtreme_dsp_slice=off  use_streaming_interface=on  has_aclken=off  has_aresetn=on  has_dout_tready=off  trim_axipin_name=on  gui_behaviour=Sysgen_GUI  input_data_width=18  ip_name=CIC Compiler  ip_version=4.0  dsptool_ready=true  wrapper_available=true  port_translation_map={ 'aclken' => 'en', 'aresetn' => 'rst' }  ipcore_xco_need_fpga_part=true  ipcore_verbose=false  block_type=cic_compiler_v4_0
  CIC Compiler 4.0 1 : xbsIndex_r4/CIC Compiler 4.0   filter_type=Decimation  number_of_stages=3  differential_delay=1  number_of_channels=1  sample_rate_changes=Fixed  fixed_or_initial_rate=16  minimum_rate=16  maximum_rate=16  ratespecification=Sample_Period  sampleperiod=1  hardwareoversamplingrate=1  quantization=Truncation  output_data_width=20  use_xtreme_dsp_slice=off  use_streaming_interface=on  has_aclken=off  has_aresetn=on  has_dout_tready=off  trim_axipin_name=on  gui_behaviour=Sysgen_GUI  input_data_width=18  ip_name=CIC Compiler  ip_version=4.0  dsptool_ready=true  wrapper_available=true  port_translation_map={ 'aclken' => 'en', 'aresetn' => 'rst' }  ipcore_xco_need_fpga_part=true  ipcore_verbose=false  block_type=cic_compiler_v4_0
  "Complex Multiplier 6.0 " : xbsIndex_r4/Complex Multiplier 6.0   hasatlast=off  hasatuser=off  atuserwidth=1  hasbtlast=off  hasbtuser=off  btuserwidth=1  multtype=Use_Mults  optimizegoal=Resources  flowcontrol=NonBlocking  outputwidth=18  roundmode=Truncate  hasctrltlast=off  hasctrltuser=off  ctrltuserwidth=1  outtlastbehv=Null  latencyconfig=Automatic  minimumlatency=37  aclken=off  aresetn=off  trim_axipin_name=on  simulation_type=hybrid_sim  simulation_model=sysgen:cmpy_v6_0  data_path_portlist={ 's_axis_a_tdata_real', 's_axis_a_tdata_imag', 's_axis_b_tdata_real', 's_axis_b_tdata_imag', 's_axis_ctrl_tdata_rounding_bit', 'm_axis_dout_tdata_real', 'm_axis_dout_tdata_imag' }  aportwidth=63  bportwidth=63  ip_name=Complex Multiplier  ip_version=6.0  dsptool_ready=true  ipcore_usecache=true  ipcore_useipmodelcache=true  ipcore_verbose=false  ipcore_latency_parameter='minimumlatency'  wrapper_available=true  port_translation_map={ 'aclken' => 'en', 'aresetn' => 'rst'}  block_type=cmpy_v6_0
  Complex Multiplier 6.0 4 : xbsIndex_r4/Complex Multiplier 6.0   hasatlast=off  hasatuser=off  atuserwidth=1  hasbtlast=off  hasbtuser=off  btuserwidth=1  multtype=Use_Mults  optimizegoal=Resources  flowcontrol=NonBlocking  outputwidth=19  roundmode=Truncate  hasctrltlast=off  hasctrltuser=off  ctrltuserwidth=1  outtlastbehv=Null  latencyconfig=Manual  minimumlatency=6  aclken=off  aresetn=off  trim_axipin_name=on  simulation_type=hybrid_sim  simulation_model=sysgen:cmpy_v6_0  data_path_portlist={ 's_axis_a_tdata_real', 's_axis_a_tdata_imag', 's_axis_b_tdata_real', 's_axis_b_tdata_imag', 's_axis_ctrl_tdata_rounding_bit', 'm_axis_dout_tdata_real', 'm_axis_dout_tdata_imag' }  aportwidth=63  bportwidth=63  ip_name=Complex Multiplier  ip_version=6.0  dsptool_ready=true  ipcore_usecache=true  ipcore_useipmodelcache=true  ipcore_verbose=false  ipcore_latency_parameter='minimumlatency'  wrapper_available=true  port_translation_map={ 'aclken' => 'en', 'aresetn' => 'rst'}  block_type=cmpy_v6_0
  Complex to Magnitude-Angle : ComplexToMagnitudeAngle  Output=Magnitude
  Constant : xbsIndex_r4/Constant  const=1  gui_display_data_type=Boolean  arith_type=Boolean  n_bits=16  bin_pt=14  preci_type=Single  exp_width=8  frac_width=24  explicit_period=off  period=1  equ=P=C  opselect=C  inp2=PCIN>>17  opr=+  inp1=P  carry=CIN  dbl_ovrd=off  block_type=constant
  Constant1 : xbsIndex_r4/Constant  const=0  gui_display_data_type=Fixed-point  arith_type=Unsigned  n_bits=16  bin_pt=16  preci_type=Single  exp_width=8  frac_width=24  explicit_period=off  period=1  equ=P=C  opselect=C  inp2=PCIN>>17  opr=+  inp1=P  carry=CIN  dbl_ovrd=off  block_type=constant
  Constant2 : xbsIndex_r4/Constant  const=0  gui_display_data_type=Fixed-point  arith_type=Unsigned  n_bits=16  bin_pt=16  preci_type=Single  exp_width=8  frac_width=24  explicit_period=off  period=1  equ=P=C  opselect=C  inp2=PCIN>>17  opr=+  inp1=P  carry=CIN  dbl_ovrd=off  block_type=constant
  Convert : xbsIndex_r4/Convert  gui_display_data_type=Fixed-point  arith_type="Signed  (2's comp)"  n_bits=16  bin_pt=14  float_type=Single  exp_bits=8  fraction_bits=24  quantization=Truncate  overflow=Saturate  en=off  latency=1  pipeline=off  dbl_ovrd=off  block_type=convert
  Convert1 : xbsIndex_r4/Convert  gui_display_data_type=Fixed-point  arith_type="Signed  (2's comp)"  n_bits=16  bin_pt=14  float_type=Single  exp_bits=8  fraction_bits=24  quantization=Truncate  overflow=Saturate  en=off  latency=1  pipeline=off  dbl_ovrd=off  block_type=convert
  Counter : xbsIndex_r4/Counter  Commented=on  cnt_type=Free Running  cnt_to=Inf  operation=Up  start_count=0  cnt_by_val=2^-8  arith_type=Unsigned  n_bits=8  bin_pt=8  load_pin=off  rst=on  en=off  explicit_period=off  period=1  use_behavioral_HDL=off  implementation=Fabric  dbl_ovrd=off  block_type=counter
  "DDS Compiler 6.0 " : xbsIndex_r4/DDS Compiler 6.0   partspresent=Phase_Generator_and_SIN_COS_LUT  dds_clock_rate=Fclk/1e6  channels=1  mode_of_operation=Standard  modulus=9  parameter_entry=Hardware_Parameters  spurious_free_dynamic_range=45  frequency_resolution=0.4  noise_shaping=None  phase_width=freqBits  output_width=IQbits  output_selection=Sine_and_Cosine  negative_sine=off  negative_cosine=off  amplitude_mode=Unit_Circle  memory_type=Auto  optimization_goal=Speed  dsp48_use=Maximal  resync=off  latency_configuration=Configurable  latency=15  has_phase_out=on  has_aclken=off  has_aresetn=off  explicit_period=on  period=Tclk  data_has_tlast=Not_Required  has_tready=off  s_phase_has_tuser=Not_Required  m_data_has_tuser=Not_Required  m_phase_has_tuser=Not_Required  s_phase_tuser_width=1  output_form=Twos_Complement  s_config_sync_mode=On_Vector  phase_increment=Programmable  output_frequency1=0  output_frequency2=0  output_frequency3=0  output_frequency4=0  output_frequency5=0  output_frequency6=0  output_frequency7=0  output_frequency8=0  output_frequency9=0  output_frequency10=0  output_frequency11=0  output_frequency12=0  output_frequency13=0  output_frequency14=0  output_frequency15=0  output_frequency16=0  pinc1='0'  pinc2='0'  pinc3='0'  pinc4='0'  pinc5='0'  pinc6='0'  pinc7='0'  pinc8='0'  pinc9='0'  pinc10='0'  pinc11='0'  pinc12='0'  pinc13='0'  pinc14='0'  pinc15='0'  pinc16='0'  phase_offset=None  phase_offset_angles1=0  phase_offset_angles2=0  phase_offset_angles3=0  phase_offset_angles4=0  phase_offset_angles5=0  phase_offset_angles6=0  phase_offset_angles7=0  phase_offset_angles8=0  phase_offset_angles9=0  phase_offset_angles10=0  phase_offset_angles11=0  phase_offset_angles12=0  phase_offset_angles13=0  phase_offset_angles14=0  phase_offset_angles15=0  phase_offset_angles16=0  poff1='0'  poff2='0'  poff3='0'  poff4='0'  poff5='0'  poff6='0'  poff7='0'  poff8='0'  poff9='0'  poff10='0'  poff11='0'  poff12='0'  poff13='0'  poff14='0'  poff15='0'  poff16='0'  trim_axipin_name=on  simulation_type=hybrid_sim  simulation_model=sysgen:xddsv6_0_cmodel  data_path_portlist={ 's_axis_config_tdata_poff', 's_axis_config_tdata_chan0_poff', 's_axis_config_tdata_pinc', 's_axis_config_tdata_chan0_pinc', 's_axis_phase_tdata_resync', 's_axis_phase_tdata_chan0_resync', 's_axis_phase_tdata_poff', 's_axis_phase_tdata_chan0_poff', 's_axis_phase_tdata_pinc', 's_axis_phase_tdata_chan0_pinc', 's_axis_phase_tdata_phase_in', 'm_axis_data_tdata_sine', 'm_axis_data_tdata_chan0_sine', 'm_axis_data_tdata_cosine', 'm_axis_data_tdata_chan0_cosine', 'm_axis_phase_tdata_phase_out', 'm_axis_phase_tdata_chan0_phase_out'}  por_mode=false  gui_behaviour=Sysgen  ip_name=DDS Compiler  ip_version=6.0  dsptool_ready=true  wrapper_available=true  port_translation_map={ 'aclken' => 'en', 'aresetn' => 'rst' }  ipcore_usecache=true  ipcore_useipmodelcache=true  ipcore_xco_need_fpga_part=true  ipcore_fpga_part=xlipgetpartsetting(gcb, {'kintex7', 'xc7k325t', '-3', 'fbg676'})  ipcore_verbose=false  block_type=dds_compiler_v6_0
  Delay : xbsIndex_r4/Delay  rst=off  infoeditControl=Selection of Reset will increase slice count due to use of real FFs and instead of SRLs  en=off  latency=6  reg_retiming=off  dbl_ovrd=off  block_type=delay
  Delay1 : xbsIndex_r4/Delay  rst=off  infoeditControl=Selection of Reset will increase slice count due to use of real FFs and instead of SRLs  en=off  latency=6  reg_retiming=off  dbl_ovrd=off  block_type=delay
  Delay2 : xbsIndex_r4/Delay  rst=off  infoeditControl=Selection of Reset will increase slice count due to use of real FFs and instead of SRLs  en=off  latency=1  reg_retiming=off  dbl_ovrd=off  block_type=delay
  Delay3 : xbsIndex_r4/Delay  rst=off  infoeditControl=Selection of Reset will increase slice count due to use of real FFs and instead of SRLs  en=off  latency=1  reg_retiming=off  dbl_ovrd=off  block_type=delay
  Delay4 : xbsIndex_r4/Delay  rst=off  infoeditControl=Selection of Reset will increase slice count due to use of real FFs and instead of SRLs  en=off  latency=2  reg_retiming=on  dbl_ovrd=off  block_type=delay
  Delay5 : xbsIndex_r4/Delay  rst=off  infoeditControl=Selection of Reset will increase slice count due to use of real FFs and instead of SRLs  en=off  latency=2  reg_retiming=on  dbl_ovrd=off  block_type=delay
  Delay6 : xbsIndex_r4/Delay  rst=off  infoeditControl=Selection of Reset will increase slice count due to use of real FFs and instead of SRLs  en=off  latency=2  reg_retiming=on  dbl_ovrd=off  block_type=delay
  Gateway Out21 : xbsIndex_r4/Gateway Out  Commented=on  inherit_from_input=off  hdl_port=off  rows=1  columns=1  UseAsDAC=off  DACChannel='1'  interface=None  automatic_assignment=on  address_offset=hex2dec('00')  intf_name=''  intf_description=''  timing_constraint=None  locs_specified=off  LOCs={}  io_standard={}  block_type=gatewayout
  Gateway Out22 : xbsIndex_r4/Gateway Out  Commented=on  inherit_from_input=off  hdl_port=off  rows=1  columns=1  UseAsDAC=off  DACChannel='1'  interface=None  automatic_assignment=on  address_offset=hex2dec('00')  intf_name=''  intf_description=''  timing_constraint=None  locs_specified=off  LOCs={}  io_standard={}  block_type=gatewayout
  Gateway Out3 : xbsIndex_r4/Gateway Out  inherit_from_input=off  hdl_port=off  rows=1  columns=1  UseAsDAC=off  DACChannel='1'  interface=None  automatic_assignment=on  address_offset=hex2dec('00')  intf_name=''  intf_description=''  timing_constraint=None  locs_specified=off  LOCs={}  io_standard={}  block_type=gatewayout
  Gateway Out4 : xbsIndex_r4/Gateway Out  inherit_from_input=off  hdl_port=off  rows=1  columns=1  UseAsDAC=off  DACChannel='1'  interface=None  automatic_assignment=on  address_offset=hex2dec('00')  intf_name=''  intf_description=''  timing_constraint=None  locs_specified=off  LOCs={}  io_standard={}  block_type=gatewayout
  Inverter : xbsIndex_r4/Inverter  Commented=on  en=off  latency=0  dbl_ovrd=off  block_type=inv
  Inverter1 : xbsIndex_r4/Inverter  en=off  latency=1  dbl_ovrd=off  block_type=inv
  Logical : xbsIndex_r4/Logical  logical_function=AND  inputs=2  en=off  latency=1  precision=Full  arith_type=Unsigned  n_bits=16  bin_pt=0  align_bp=on  dbl_ovrd=off  block_type=logical
  Mult{1..2,8..9} (4 alike) : xbsIndex_r4/Mult  precision=User Defined  arith_type="Signed  (2's comp)"  n_bits=16  bin_pt=15  quantization=Truncate  overflow=Wrap  en=off  latency=3  use_behavioral_HDL=off  opt=Speed  use_embedded=on  optimum_pipeline=off  pipeline=on  dbl_ovrd=off  use_rpm=on  placement_style=Triangular  block_type=mult
  Mux13 : xbsIndex_r4/Mux  inputs=2  en=off  latency=0  precision=Full  arith_type=Unsigned  n_bits=16  bin_pt=14  quantization=Truncate  overflow=Wrap  dbl_ovrd=off  block_type=mux
  Mux4 : Mux  Inputs=3
  Real-Imag to Complex : RealImagToComplex
  Register : xbsIndex_r4/Register  init=0  rst=off  en=on  dbl_ovrd=off  block_type=register
  Register1 : xbsIndex_r4/Register  init=0  rst=off  en=on  dbl_ovrd=off  block_type=register
  Register2 : xbsIndex_r4/Register  init=0  rst=off  en=on  dbl_ovrd=off  block_type=register
  Register{3..6} (4 alike) : xbsIndex_r4/Register  init=0  rst=off  en=off  dbl_ovrd=off  block_type=register
  Relational : xbsIndex_r4/Relational  mode=a=b  op_type=Bool  en=off  latency=1  dbl_ovrd=off  block_type=relational
  Relational1 : xbsIndex_r4/Relational  mode=a=b  op_type=Bool  en=off  latency=0  dbl_ovrd=off  block_type=relational
  Relational2 : xbsIndex_r4/Relational  mode=a!=b  op_type=Ufix  en=off  latency=1  dbl_ovrd=off  block_type=relational
  Relational3 : xbsIndex_r4/Relational  mode=a!=b  op_type=Bool  en=off  latency=0  dbl_ovrd=off  block_type=relational
  Scale1 : xbsIndex_r4/Scale  scale_factor=-12  dbl_ovrd=off  block_type=scale
  Scale2 : xbsIndex_r4/Scale  scale_factor=-12  dbl_ovrd=off  block_type=scale
  Terminator{,1..3,8} (5 alike) : Terminator
  block downconverter Scope : Scope
  block downconverter Scope1 : Scope  Commented=on  NumInputPorts=2
  demod : Outport
  toDAC : Outport  Port=2
  freq : Outport  Port=3
  DDS phase : Outport  Port=4
  wires:
  Relational/1 -> Logical/1, Inverter1/1
  Bus Selector1/1 -> Relational/2  "<channel>"
  Bus Selector1/2 -> Delay4/1  "<freq>"
  addrIn/1 -> Relational1/1, Relational/1, [Addr]
  "DDS Compiler 6.0 "/2 -> Complex Multiplier 6.0 4/2, Delay/1
  "DDS Compiler 6.0 "/3 -> Complex Multiplier 6.0 4/3, Delay1/1
  In/1 -> Bus Selector2/1
  Relational1/1 -> Register1/2, Register/2
  Register1/1 -> Complex Multiplier 6.0 4/6
  Register/1 -> Relational2/2, Complex Multiplier 6.0 4/5
  "DDS Compiler 6.0 "/1 -> Complex Multiplier 6.0 4/1, Complex Multiplier 6.0 4/4
  Delay/1 -> Delay2/1
  Delay1/1 -> Delay3/1
  [sin0] -> "Complex Multiplier 6.0 "/2
  [cos0] -> "Complex Multiplier 6.0 "/3
  "Complex Multiplier 6.0 "/2 -> "CIC Compiler 4.0 "/2
  "CIC Compiler 4.0 "/3 -> Scale1/1
  CIC Compiler 4.0 1/3 -> Scale2/1
  "Complex Multiplier 6.0 "/1 -> "CIC Compiler 4.0 "/1, CIC Compiler 4.0 1/1
  "CIC Compiler 4.0 "/1 -> Terminator/1
  CIC Compiler 4.0 1/1 -> Terminator2/1
  CIC Compiler 4.0 1/2 -> Terminator3/1
  Complex Multiplier 6.0 4/1 -> Terminator8/1
  Bus Creator/1 -> toDAC/1
  Bus Selector/2 -> Register/1  "<dPhiQ>"
  Bus Selector/3 -> Register1/1  "<dPhiI>"
  [dphiBus] -> Bus Selector/1
  Bus Selector/1 -> Relational1/2  "<channel>"
  Complex Multiplier 6.0 4/3 -> Convert/1
  Complex Multiplier 6.0 4/2 -> Convert1/1
  Constant1/1 -> Mux13/2
  [Ampl0] -> Mux13/3
  Mux13/1 -> Mult2/2, Mult9/2, Mult1/2, Mult8/2
  Constant2/1 -> Relational2/1
  Relational2/1 -> Mux13/1
  Relational3/1 -> Inverter/1, CIC Compiler 4.0 1/3, "CIC Compiler 4.0 "/3
  [Addr] -> Relational3/2
  synchIn/1 -> Relational3/1
  "CIC Compiler 4.0 "/2 -> Terminator1/1
  [freqBusHBW] -> Bus Selector1/1
  Convert1/1 -> Mult9/1
  Delay3/1 -> [sin0], Mult8/1
  Delay2/1 -> Mult1/1, [cos0]
  Delay4/1 -> Register2/1, "DDS Compiler 6.0 "/2
  Inverter1/1 -> Logical/2
  Logical/1 -> Register2/2, "DDS Compiler 6.0 "/1
  "Complex Multiplier 6.0 "/3 -> CIC Compiler 4.0 1/2
  Constant/1 -> "Complex Multiplier 6.0 "/4, "Complex Multiplier 6.0 "/1
  Convert/1 -> Mult2/1
  Mult2/1 -> Register6/1  "I1"
  Mult9/1 -> Register5/1  "Q1"
  Mult8/1 -> Register4/1  "I0"
  Mult1/1 -> Register3/1  "Q0"
  Bus Creator1/1 -> demod/1
  Scale1/1 -> Gateway Out3/1, Bus Creator1/1  "Q"
  Scale2/1 -> Gateway Out4/1, Bus Creator1/2  "I"
  Gateway Out4/1 -> Mux4/2, Real-Imag to Complex/1
  Gateway Out3/1 -> Mux4/1, Real-Imag to Complex/2
  Mux4/1 -> block downconverter Scope/1
  Gateway Out22/1 -> block downconverter Scope1/2
  Complex to Magnitude-Angle/1 -> Mux4/3
  Gateway Out21/1 -> block downconverter Scope1/1
  Counter/1 -> Gateway Out22/1
  Inverter/1 -> Counter/1, Gateway Out21/1
  Real-Imag to Complex/1 -> Complex to Magnitude-Angle/1
  Register2/1 -> freq/1, [freq]
  Delay6/1 -> "Complex Multiplier 6.0 "/6
  Delay5/1 -> "Complex Multiplier 6.0 "/5
  Register3/1 -> Bus Creator/1  "Q0"
  Register4/1 -> Bus Creator/2  "I0"
  Register5/1 -> Bus Creator/3  "Q1"
  Register6/1 -> Bus Creator/4  "I1"
  "DDS Compiler 6.0 "/5 -> DDS phase/1
  Bus Selector2/2 -> Delay6/1  "<freq>"
  Bus Selector2/1 -> Delay5/1  "<channel>"
